simulink model "EV_Powertrain_Simulation"  (R2025a)
settings: Solver=VariableStepAuto  StartTime=0.0  StopTime=100  RelTol=1e-3
values from neighbouring files (symbols this model uses):
  air_density = 1.225    [EV_Parameters.m]
  battery_capacity_Ah = 75    [EV_Parameters.m]
  battery_voltage = 400    [EV_Parameters.m]
  Crr = 0.015    [EV_Parameters.m]
  drag_coefficient = 0.28    [EV_Parameters.m]
  F_grade = vehicle_mass * g * sind(road_grade)    [EV_Parameters.m]
  frontal_area = 2.2    [EV_Parameters.m]
  g = 9.81    [EV_Parameters.m]
  gear_efficiency = 0.95    [EV_Parameters.m]
  gear_ratio = 9    [EV_Parameters.m]
  initial_soc = 90    [EV_Parameters.m]
  Kd = 0    [EV_Parameters.m]
  Ki = 10    [EV_Parameters.m]
  Kp = 60    [EV_Parameters.m]
  motor_efficiency = 0.95    [EV_Parameters.m]
  motor_max_torque = 250    [EV_Parameters.m]
  vehicle_mass = 1500    [EV_Parameters.m]
  wheel_radius = 0.30    (= 0.3)    [EV_Parameters.m]
libraries: simulink x1, slpidlib x1
settings Model: Creator=rajes  LastModifiedBy=rajes

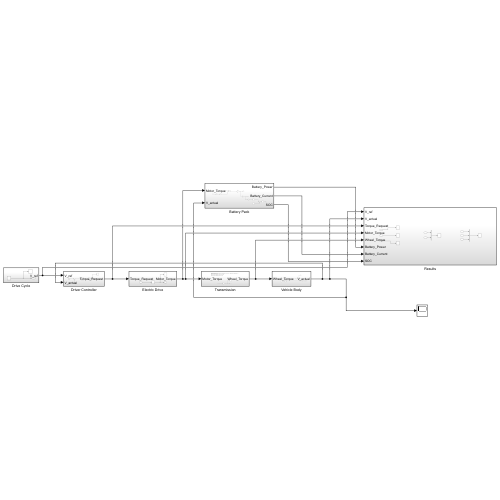
[thumbnail: Simulink's stored preview of the top-level diagram]
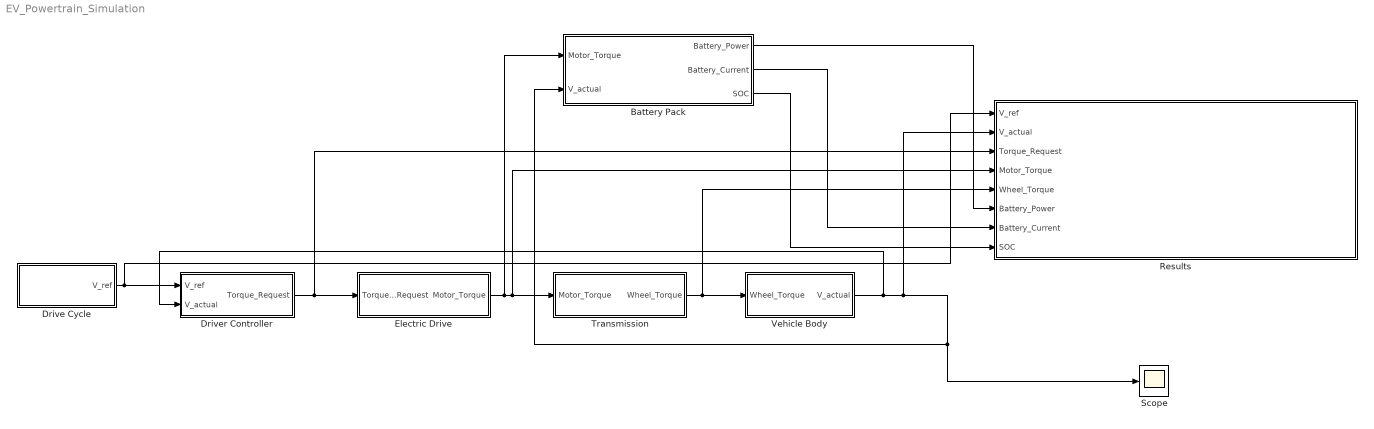
== system EV_Powertrain_Simulation ==
  Battery Pack : Subsystem
  Drive Cycle : Subsystem
  Driver Controller : Subsystem
  Electric Drive : Subsystem
  Results : Subsystem
  Scope : Scope
      settings: ActiveDisplayYMinimum=-2.0807768461578782  ActiveDisplayYMaximum=18.378466100825083  DataLoggingVariableName=ScopeData5
  Transmission : Subsystem
  Vehicle Body : Subsystem
  wires:
  Drive Cycle/1(V_ref) -> Results/1(V_ref), Driver Controller/1(V_ref)
  Driver Controller/1(Torque_Request) -> Results/3(Torque_Request), Electric Drive/1(Torque_Request)
  Electric Drive/1(Motor_Torque) -> Battery Pack/1(Motor_Torque), Results/4(Motor_Torque), Transmission/1(Motor_Torque)
  Transmission/1(Wheel_Torque) -> Results/5(Wheel_Torque), Vehicle Body/1(Wheel_Torque)
  Vehicle Body/1(V_actual) -> Driver Controller/2(V_actual), Results/2(V_actual), Scope/1, Battery Pack/2(V_actual)
  Battery Pack/1(Battery_Power) -> Results/6(Battery_Power)
  Battery Pack/2(Battery_Current) -> Results/7(Battery_Current)
  Battery Pack/3(SOC) -> Results/8(SOC)

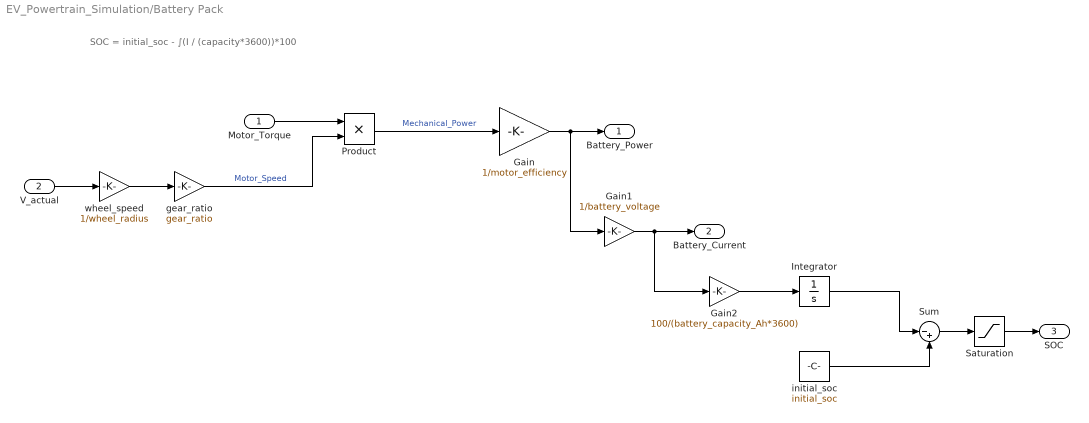
== system EV_Powertrain_Simulation/Battery Pack ==
  note: SOC = initial_soc - ∫(I / (capacity*3600))*100
  Motor_Torque : Inport
  V_actual : Inport  Port=2
  Gain : Gain  Gain=1/motor_efficiency
  Gain1 : Gain  Gain=1/battery_voltage
  Gain2 : Gain  Gain=100/(battery_capacity_Ah*3600)
  Integrator : Integrator
  Product : Product
  Saturation : Saturate  UpperLimit=100  LowerLimit=0
  Sum : Sum  Inputs=|-+
  gear_ratio : Gain  Gain=gear_ratio
  initial_soc : Constant  Value=initial_soc
  wheel_speed : Gain  Gain=1/wheel_radius
  Battery_Power : Outport
  Battery_Current : Outport  Port=2
  SOC : Outport  Port=3
  wires:
  V_actual/1 -> wheel_speed/1
  wheel_speed/1 -> gear_ratio/1
  Motor_Torque/1 -> Product/1
  gear_ratio/1 -> Product/2  "Motor_Speed"
  Product/1 -> Gain/1  "Mechanical_Power"
  Gain/1 -> Gain1/1, Battery_Power/1
  Gain1/1 -> Gain2/1, Battery_Current/1
  Gain2/1 -> Integrator/1
  Integrator/1 -> Sum/1
  initial_soc/1 -> Sum/2
  Sum/1 -> Saturation/1
  Saturation/1 -> SOC/1

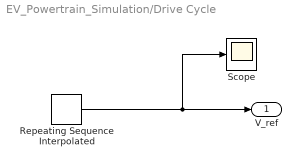
== system EV_Powertrain_Simulation/Drive Cycle ==
  Repeating Sequence Interpolated : simulink/Sources/Repeating Sequence Interpolated  OutValues=[0 8.3 16.7 16.7 0 0]  TimeValues=[0 10 30 60 80 100]  LookUpMeth=Interpolation-Use End Values  tsamp=0.01  OutMin=[]  OutMax=[]  OutDataTypeStr=double  OutputDataTypeScalingMode=double  OutDataType=fixdt(0,8)  OutScaling=2^-10
  Scope : Scope
      settings: ActiveDisplayYMinimum=-194.8349481414574  ActiveDisplayYMaximum=160.79378387416295
  V_ref : Outport
  wires:
  Repeating Sequence Interpolated/1 -> Scope/1, V_ref/1

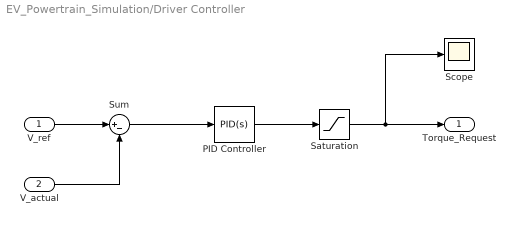
== system EV_Powertrain_Simulation/Driver Controller ==
  V_ref : Inport
  V_actual : Inport  Port=2
  PID Controller : slpidlib/PID Controller  Controller=PID  Form=Parallel  TimeDomain=Continuous-time  UseExternalTs=off  SampleTime=-1  IntegratorMethod=Forward Euler  FilterMethod=Forward Euler  ControllerParametersSource=internal  P=Kp  I=Ki  UseKiTs=off  D=Kd  UseExternalDerivativeSource=off  N=100  UseFilter=on  TunerSelectOption=Transfer Function Based (PID Tuner App)  InitialConditionSource=internal  InitialConditionForIntegrator=0  InitialConditionForFilter=0  DifferentiatorICPrevScaledInput=0  ExternalReset=none  TrackingMode=off  Kt=1  LimitOutput=off  SatLimitsSource=internal  UpperSaturationLimit=inf  LowerSaturationLimit=-inf  LinearizeAsGain=on  AntiWindupMode=none  Kb=1  LimitIntegrator=off  UpperIntegratorSaturationLimit=inf  LowerIntegratorSaturationLimit=-inf  POutMin=[]  POutMax=[]  IOutMin=[]  IOutMax=[]  DOutMin=[]  DOutMax=[]  NOutMin=[]  NOutMax=[]  SumOutMin=[]  SumOutMax=[]  SaturationOutMin=[]  SaturationOutMax=[]  PParamMin=[]  PParamMax=[]  IParamMin=[]  IParamMax=[]  DParamMin=[]  DParamMax=[]  NParamMin=[]  NParamMax=[]  KbParamMin=[]  KbParamMax=[]  KtParamMin=[]  KtParamMax=[]  KbOutMin=[]  KbOutMax=[]  KtOutMin=[]  KtOutMax=[]  IntegratorOutMin=[]  IntegratorOutMax=[]  FilterOutMin=[]  FilterOutMax=[]  SumI1OutMin=[]  SumI1OutMax=[]  SumI2OutMin=[]  SumI2OutMax=[]  SumI3OutMin=[]  SumI3OutMax=[]  SumI4OutMin=[]  SumI4OutMax=[]  SumDOutMin=[]  SumDOutMax=[]  DifferentiatorOutMin=[]  DifferentiatorOutMax=[]  FilterDiffOutCoefMin=[]  FilterDiffOutCoefMax=[]  ReciprocalOutMin=[]  ReciprocalOutMax=[]  SumDenOutMin=[]  SumDenOutMax=[]  SumNumOutMin=[]  SumNumOutMax=[]  DivideOutMin=[]  DivideOutMax=[]  UdiffTsProdOutMin=[]  UdiffTsProdOutMax=[]  NTsProdOutMin=[]  NTsProdOutMax=[]  UintegralTsProdOutMin=[]  UintegralTsProdOutMax=[]  UngainTsProdOutMin=[]  UngainTsProdOutMax=[]  ClampingZeroOutDataTypeStr=Inherit: Inherit via back propagation  ClampingZeroOutMin=[]  ClampingZeroOutMax=[]  FilterDenConstantOutDataTypeStr=Inherit: Inherit via back propagation  FilterDenConstantOutMin=[]  FilterDenConstantOutMax=[]  PCopyOutDataTypeStr=Inherit: Inherit via back propagation  PCopyOutMin=[]  PCopyOutMax=[]  NCopyOutDataTypeStr=Inherit: Inherit via back propagation  NCopyOutMin=[]  NCopyOutMax=[]  IntegratorContinuousStateAttributes=''  IntegratorStateMustResolveToSignalObject=off  IntegratorRTWStateStorageClass=Auto  FilterContinuousStateAttributes=''  FilterStateMustResolveToSignalObject=off  FilterRTWStateStorageClass=Auto  ParallelPVariant=InternalParameters  IdealPVariant=Disabled  IVariant=InternalParameters  DVariant=InternalParameters  IntegratorVariant=Continuous  SatVariant=Disabled  AWVariant=Passthrough  PCopyVariant=Disabled  TRVariant=Disabled  FdbkBlocksVariant=Forward  IdealPFdbkVariant=Disabled  SatFdbkVariant=Disabled  DerivativeFilterVariant=ContFilter  NVariant=InternalParameters  NCopyVariant=Disabled  FilterICVariant=InternalICsFilter  IntegratorICVariant=InternalICs  ExternalResetVariant=Disabled  TRSumVariant=Passthrough  SumFdbkVariant=Disabled  SumVariant=Sum_PID  TsampFilterVariant=InternalTs  TsampNgainVariant=Passthrough  TsampIntegralVariant=Disabled_SignalSpec  ExternalSaturationOutDataTypeStr=Inherit: Same as second input  DerivativeSourceVariant=ErrorSignal  PreIntVariant=InternalPreInt
  Saturation : Saturate  UpperLimit=250  LowerLimit=-120
  Scope : Scope
      settings: ActiveDisplayYMinimum=-144.79711923637353  ActiveDisplayYMaximum=334.10467674188772
  Sum : Sum  Inputs=|+-
  Torque_Request : Outport
  wires:
  V_ref/1 -> Sum/1
  V_actual/1 -> Sum/2
  Sum/1 -> PID Controller/1
  PID Controller/1 -> Saturation/1
  Saturation/1 -> Scope/1, Torque_Request/1

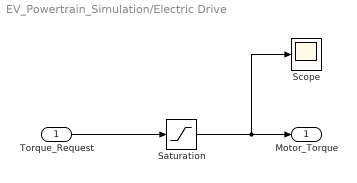
== system EV_Powertrain_Simulation/Electric Drive ==
  Torque_Request : Inport
  Saturation : Saturate  UpperLimit=motor_max_torque  LowerLimit=-motor_max_torque
  Scope : Scope
      settings: ActiveDisplayYMinimum=-1  ActiveDisplayYMaximum=1  DataLoggingVariableName=ScopeData2
  Motor_Torque : Outport
  wires:
  Torque_Request/1 -> Saturation/1
  Saturation/1 -> Scope/1, Motor_Torque/1

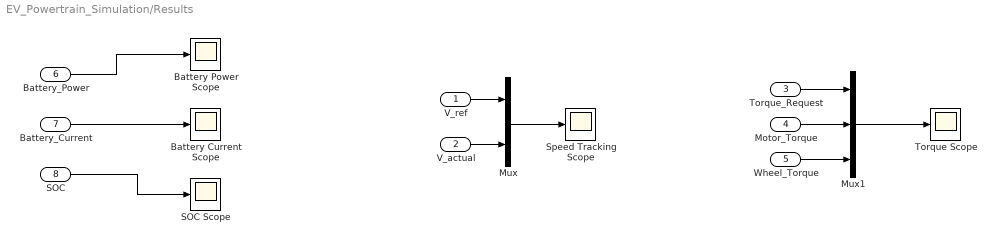
== system EV_Powertrain_Simulation/Results ==
  V_ref : Inport
  V_actual : Inport  Port=2
  Torque_Request : Inport  Port=3
  Motor_Torque : Inport  Port=4
  Wheel_Torque : Inport  Port=5
  Battery_Power : Inport  Port=6
  Battery_Current : Inport  Port=7
  SOC : Inport  Port=8
  Battery Current Scope : Scope
      settings: ActiveDisplayYMinimum=-57.652458372550392  ActiveDisplayYMaximum=70.561363103829734  DataLoggingVariableName=ScopeData9
  Battery Power Scope : Scope
      settings: ActiveDisplayYMinimum=-43514.140443063072  ActiveDisplayYMaximum=7078.6860994752478  DataLoggingVariableName=ScopeData8
  Mux : Mux  Inputs=2
  Mux1 : Mux  Inputs=3
  SOC Scope : Scope
      settings: ActiveDisplayYMinimum=88.373114815343442  ActiveDisplayYMaximum=90.447622616263459  DataLoggingVariableName=ScopeData10
  Speed Tracking Scope : Scope
      settings: ActiveDisplayYMinimum=-2.7575287498109873  ActiveDisplayYMaximum=19.17904253944447  DataLoggingVariableName=ScopeData6
  Torque Scope : Scope
      settings: ActiveDisplayYMinimum=-806.221502628334  ActiveDisplayYMaximum=163.08302020627326  DataLoggingVariableName=ScopeData7
  wires:
  V_ref/1 -> Mux/1
  V_actual/1 -> Mux/2
  Mux/1 -> Speed Tracking Scope/1
  Torque_Request/1 -> Mux1/1
  Motor_Torque/1 -> Mux1/2
  Wheel_Torque/1 -> Mux1/3
  Mux1/1 -> Torque Scope/1
  Battery_Power/1 -> Battery Power Scope/1
  Battery_Current/1 -> Battery Current Scope/1
  SOC/1 -> SOC Scope/1

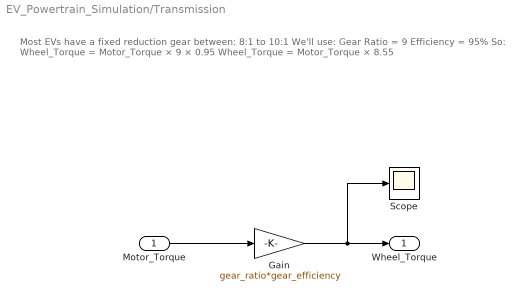
== system EV_Powertrain_Simulation/Transmission ==
  note: Most EVs have a fixed reduction gear between: 8:1 to 10:1 We'll use: Gear Ratio = 9 Efficiency = 95% So:
      | Wheel_Torque = Motor_Torque × 9 × 0.95
      | Wheel_Torque = Motor_Torque × 8.55
  Motor_Torque : Inport
  Gain : Gain  Gain=gear_ratio*gear_efficiency
  Scope : Scope
      settings: ActiveDisplayYMinimum=2094.3987382211003  ActiveDisplayYMaximum=2148.7774526342355  DataLoggingVariableName=ScopeData3
  Wheel_Torque : Outport
  wires:
  Motor_Torque/1 -> Gain/1
  Gain/1 -> Scope/1, Wheel_Torque/1

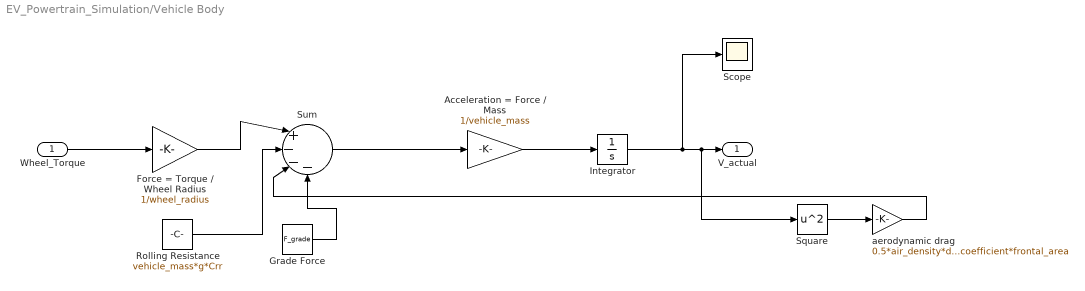
== system EV_Powertrain_Simulation/Vehicle Body ==
  Wheel_Torque : Inport
  Acceleration = Force / Mass : Gain  Gain=1/vehicle_mass
  Force = Torque / Wheel Radius : Gain  Gain=1/wheel_radius
  Grade Force : Constant  Value=F_grade
  Integrator : Integrator
  Rolling Resistance : Constant  Value=vehicle_mass*g*Crr
  Scope : Scope
      settings: ActiveDisplayYMinimum=-1  ActiveDisplayYMaximum=1  DataLoggingVariableName=ScopeData4
  Square : Math  Operator=square
  Sum : Sum  Inputs=|+---
  aerodynamic drag : Gain  Gain=0.5*air_density*drag_coefficient*frontal_area
  V_actual : Outport
  wires:
  Wheel_Torque/1 -> Force = Torque / Wheel Radius/1
  Acceleration = Force / Mass/1 -> Integrator/1
  Integrator/1 -> Scope/1, Square/1, V_actual/1
  Square/1 -> aerodynamic drag/1
  Force = Torque / Wheel Radius/1 -> Sum/1
  Rolling Resistance/1 -> Sum/2
  aerodynamic drag/1 -> Sum/3
  Sum/1 -> Acceleration = Force / Mass/1
  Grade Force/1 -> Sum/4
